simulink model "Boomerang_Simulink_Nav"  (R2023a)
settings: Solver=ode4  StartTime=0.0  StopTime=t  FixedStep=dt  MaxStep=maxstep  MinStep=minstep
values from neighbouring files (symbols this model uses):
  c = 5e-2    (= 0.05)    [Boomerang_Sim.m]
  CDdata = [x_CD, y_CD]    [Boomerang_Sim.m]
  CLdata = [x_CL, y_CL]    [Boomerang_Sim.m]
  CMdata = [x_CM, y_CM]    [Boomerang_Sim.m]
  Eul0 = [0; 0; 0]    [Boomerang_Sim.m]
  f = 1000    [Boomerang_Sim.m]
  g = 8.87    [Boomerang_Sim.m]
  invJ = inv(J)    [Boomerang_Sim.m]
  invTI0 = transpose(TI0)    [Boomerang_Sim.m]
  invTj = zeros(3,3,nw)    [Boomerang_Sim.m]
  J = J + (Ji(:,:,i))    [Boomerang_Sim.m]
  l_integrate = linspace(0,l_blade,n)    [Boomerang_Sim.m]
  m = m_b    (= 0.2)    [Boomerang_Sim.m]
  nw = 4    [Boomerang_Sim.m]
  omega0 = [0; 0; 10*pi*2]    [Boomerang_Sim.m]
  PHI0 = deg2rad(PHI0)    [Boomerang_Sim.m]
  PSI0 = deg2rad(PSI0)    [Boomerang_Sim.m]
  R_pos0 = [0; 0; 1.5]    [Boomerang_Sim.m]
  rho = 1.3288    [Boomerang_Sim.m]
  S = pi*R^2    (= 0.196349540849)    [Boomerang_Sim.m]
  THETA0 = deg2rad(THETA0)    [Boomerang_Sim.m]
  thetaj = 0    [Boomerang_Sim.m]
  TI0 = RI01*RI02*RI03    [Boomerang_Sim.m]
  Tj = zeros(3,3, nw)    [Boomerang_Sim.m]
  u0 = TI0*U0    [Boomerang_Sim.m]
  v_wind = [0; 0; 0]    [Boomerang_Sim.m]
  x_ac = zeros(3,nw)    [Boomerang_Sim.m]
undefined symbols (not defined in the file or in its folder): delta_theta, t_action
libraries: aerolibnav x2, simulink_extras x2
settings Model: Creator=dsantis  LastModifiedBy=dsantis

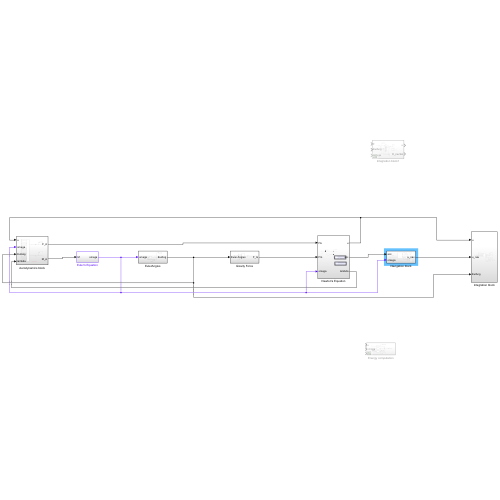
[thumbnail: Simulink's stored preview of the top-level diagram]
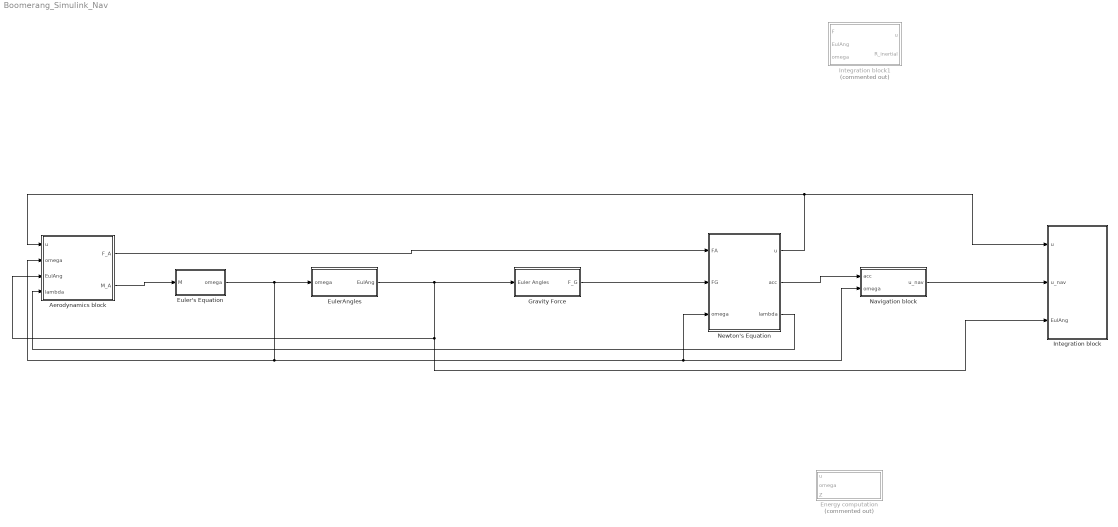
== system Boomerang_Simulink_Nav ==
  Aerodynamics block : Subsystem
  Energy computation : Subsystem  Commented=on
  Euler's Equation : Subsystem
  EulerAngles : Subsystem
  Gravity Force : Subsystem
  Integration block : Subsystem
  Integration block1 : Subsystem  Commented=on
  Navigation block : Subsystem
  Newton's Equation : Subsystem
  wires:
  Euler's Equation/1(omega) -> EulerAngles/1(omega), Aerodynamics block/2(omega), Newton's Equation/3(omega), Navigation block/2(omega)
  Newton's Equation/1(u) -> Aerodynamics block/1(u), Integration block/1(u)
  Gravity Force/1(F_G) -> Newton's Equation/2(FG)
  Aerodynamics block/2(M_A) -> Euler's Equation/1(M)
  EulerAngles/1(EulAng) -> Aerodynamics block/3(EulAng), Integration block/3(EulAng), Gravity Force/1(Euler Angles)
  Aerodynamics block/1(F_A) -> Newton's Equation/1(FA)
  Navigation block/1(u_nav) -> Integration block/2(u_nav)
  Newton's Equation/2(acc) -> Navigation block/1(acc)
  Newton's Equation/3(lambda) -> Aerodynamics block/4(lambda)

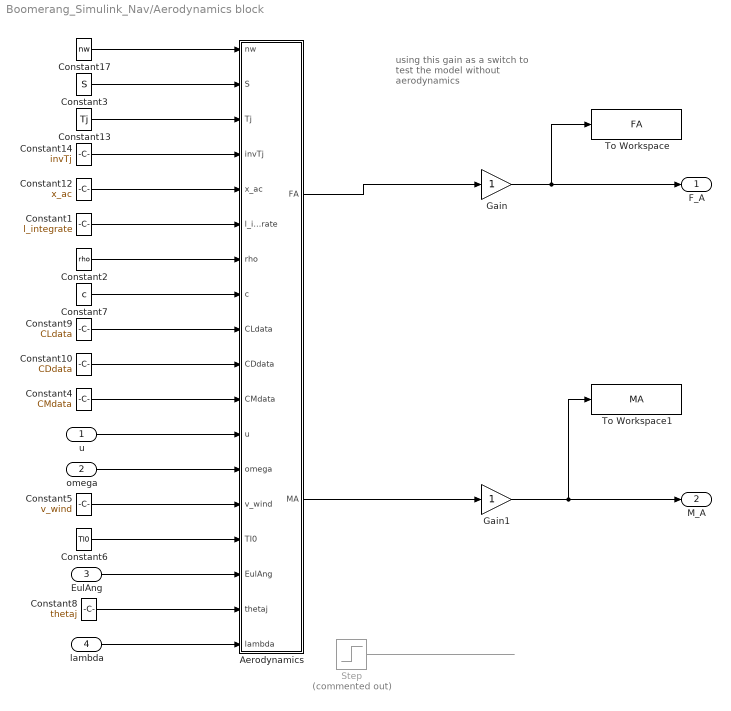
== system Boomerang_Simulink_Nav/Aerodynamics block ==
  note: using this gain as a switch
      | to test the model without aerodynamics
  u : Inport
  omega : Inport  Port=2
  EulAng : Inport  Port=3
  lambda : Inport  Port=4
  Aerodynamics : MATLAB Function  TreatAsAtomicUnit=on
  Constant1 : Constant  Value=l_integrate
  Constant10 : Constant  Value=CDdata
  Constant12 : Constant  Value=x_ac
  Constant13 : Constant  Value=Tj
  Constant14 : Constant  Value=invTj
  Constant17 : Constant  Value=nw
  Constant2 : Constant  Value=rho
  Constant3 : Constant  Value=S
  Constant4 : Constant  Value=CMdata
  Constant5 : Constant  Value=v_wind
  Constant6 : Constant  Value=TI0
  Constant7 : Constant  Value=c
  Constant8 : Constant  Value=thetaj
  Constant9 : Constant  Value=CLdata
  Gain : Gain
  Gain1 : Gain
  Step : Step  Commented=on  Time=t_action  After=delta_theta  SampleTime=0  VectorParams1D=off
  To Workspace : ToWorkspace  VariableName=FA  SampleTime=-1
  To Workspace1 : ToWorkspace  VariableName=MA  SampleTime=-1
  F_A : Outport
  M_A : Outport  Port=2
  wires:
  u/1 -> Aerodynamics/12(u)
  Constant2/1 -> Aerodynamics/7(rho)
  Constant9/1 -> Aerodynamics/9(CLdata)
  Constant10/1 -> Aerodynamics/10(CDdata)
  Constant1/1 -> Aerodynamics/6(l_integrate)
  Constant7/1 -> Aerodynamics/8(c)
  omega/1 -> Aerodynamics/13(omega)
  Constant12/1 -> Aerodynamics/5(x_ac)
  Constant14/1 -> Aerodynamics/4(invTj)
  Constant13/1 -> Aerodynamics/3(Tj)
  Aerodynamics/1(FA) -> Gain/1
  Constant17/1 -> Aerodynamics/1(nw)
  Constant3/1 -> Aerodynamics/2(S)
  Gain/1 -> To Workspace/1, F_A/1
  Constant4/1 -> Aerodynamics/11(CMdata)
  Step/1 -> ?
  Aerodynamics/2(MA) -> Gain1/1
  Constant5/1 -> Aerodynamics/14(v_wind)
  Constant6/1 -> Aerodynamics/15(TI0)
  EulAng/1 -> Aerodynamics/16(EulAng)
  Constant8/1 -> Aerodynamics/17(thetaj)
  lambda/1 -> Aerodynamics/18(lambda)
  Gain1/1 -> To Workspace1/1, M_A/1

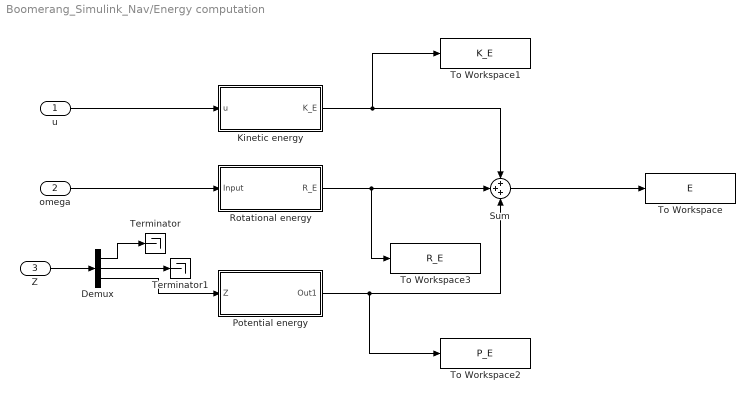
== system Boomerang_Simulink_Nav/Energy computation ==
  u : Inport
  omega : Inport  Port=2
  Z : Inport  Port=3
  Demux : Demux  Outputs=3
  Kinetic energy : Subsystem
  Potential energy : Subsystem
  Rotational energy : Subsystem
  Sum : Sum  Inputs=+++
  Terminator : Terminator
  Terminator1 : Terminator
  To Workspace : ToWorkspace  VariableName=E  SaveFormat=Timeseries  SampleTime=-1
  To Workspace1 : ToWorkspace  VariableName=K_E  SaveFormat=Timeseries  SampleTime=-1
  To Workspace2 : ToWorkspace  VariableName=P_E  SaveFormat=Timeseries  SampleTime=-1
  To Workspace3 : ToWorkspace  VariableName=R_E  SaveFormat=Timeseries  SampleTime=-1
  wires:
  u/1 -> Kinetic energy/1(u)
  omega/1 -> Rotational energy/1(Input)
  Z/1 -> Demux/1
  Demux/3 -> Potential energy/1(Z)
  Demux/1 -> Terminator/1
  Demux/2 -> Terminator1/1
  Kinetic energy/1(K_E) -> To Workspace1/1, Sum/1
  Rotational energy/1(R_E) -> To Workspace3/1, Sum/2
  Potential energy/1(Out1) -> To Workspace2/1, Sum/3
  Sum/1 -> To Workspace/1

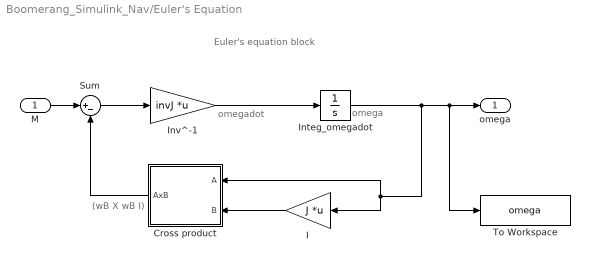
== system Boomerang_Simulink_Nav/Euler's Equation ==
  note: Euler's equation block
  note: (wB X wB I)
  note: omega
  note: omegadot
  M : Inport
  Cross product : Subsystem
  I : Gain  Gain=J  Multiplication=Matrix(K*u)
  Integ_omegadot : Integrator  InitialCondition=omega0
  Inv^-1 : Gain  Gain=invJ  Multiplication=Matrix(K*u) (u vector)
  Sum : Sum  Inputs=|+-
  To Workspace : ToWorkspace  VariableName=omega  SampleTime=-1
  omega : Outport  VectorParamsAs1DForOutWhenUnconnected=off
  wires:
  Integ_omegadot/1 -> To Workspace/1, omega/1, I/1, Cross product/1(A)
  I/1 -> Cross product/2(B)
  M/1 -> Sum/1
  Sum/1 -> Inv^-1/1
  Inv^-1/1 -> Integ_omegadot/1
  Cross product/1(AxB) -> Sum/2

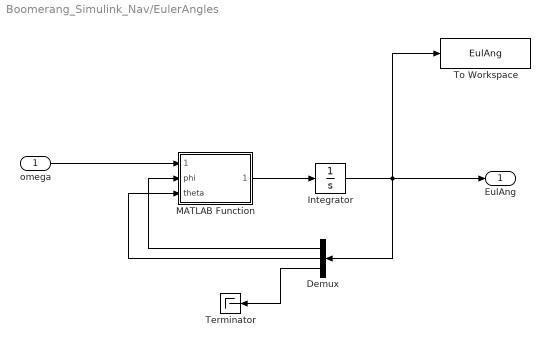
== system Boomerang_Simulink_Nav/EulerAngles ==
  omega : Inport
  Demux : Demux  Outputs=3
  Integrator : Integrator  InitialCondition=Eul0
  MATLAB Function : MATLAB Function  TreatAsAtomicUnit=on
  Terminator : Terminator
  To Workspace : ToWorkspace  VariableName=EulAng  SampleTime=-1
  EulAng : Outport
  wires:
  omega/1 -> MATLAB Function/1(omega)
  MATLAB Function/1(EulRate) -> Integrator/1
  Integrator/1 -> To Workspace/1, Demux/1, EulAng/1
  Demux/1 -> MATLAB Function/2(phi)
  Demux/2 -> MATLAB Function/3(theta)
  Demux/3 -> Terminator/1

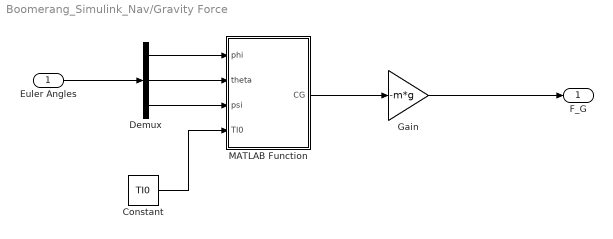
== system Boomerang_Simulink_Nav/Gravity Force ==
  Euler Angles : Inport
  Constant : Constant  Value=TI0
  Demux : Demux  Outputs=3
  Gain : Gain  Gain=-m*g
  MATLAB Function : MATLAB Function  TreatAsAtomicUnit=on
  F_G : Outport
  wires:
  Gain/1 -> F_G/1
  Demux/3 -> MATLAB Function/3(psi)
  Demux/2 -> MATLAB Function/2(theta)
  Demux/1 -> MATLAB Function/1(phi)
  MATLAB Function/1(CG) -> Gain/1
  Euler Angles/1 -> Demux/1
  Constant/1 -> MATLAB Function/4(TI0)

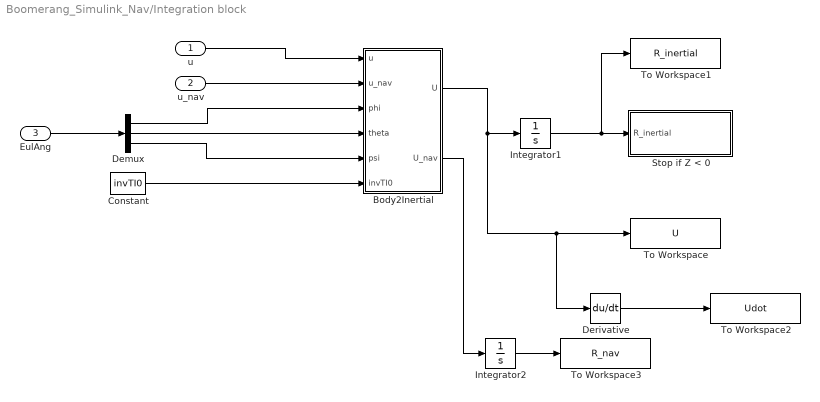
== system Boomerang_Simulink_Nav/Integration block ==
  u : Inport
  u_nav : Inport  Port=2
  EulAng : Inport  Port=3
  Body2Inertial : MATLAB Function  TreatAsAtomicUnit=on
  Constant : Constant  Value=invTI0
  Demux : Demux  Outputs=3
  Derivative : Derivative
  Integrator1 : Integrator  InitialCondition=R_pos0
  Integrator2 : Integrator  InitialCondition=R_pos0
  Stop if Z < 0 : Subsystem
  To Workspace : ToWorkspace  VariableName=U  SampleTime=-1
  To Workspace1 : ToWorkspace  VariableName=R_inertial  SampleTime=-1
  To Workspace2 : ToWorkspace  VariableName=Udot  SaveFormat=Timeseries  SampleTime=-1
  To Workspace3 : ToWorkspace  VariableName=R_nav  SampleTime=-1
  wires:
  Derivative/1 -> To Workspace2/1
  Integrator1/1 -> Stop if Z < 0/1(R_inertial), To Workspace1/1
  Body2Inertial/1(U) -> Derivative/1, To Workspace/1, Integrator1/1
  Demux/3 -> Body2Inertial/5(psi)
  Demux/2 -> Body2Inertial/4(theta)
  u/1 -> Body2Inertial/1(u)
  Demux/1 -> Body2Inertial/3(phi)
  Constant/1 -> Body2Inertial/6(invTI0)
  EulAng/1 -> Demux/1
  u_nav/1 -> Body2Inertial/2(u_nav)
  Body2Inertial/2(U_nav) -> Integrator2/1
  Integrator2/1 -> To Workspace3/1

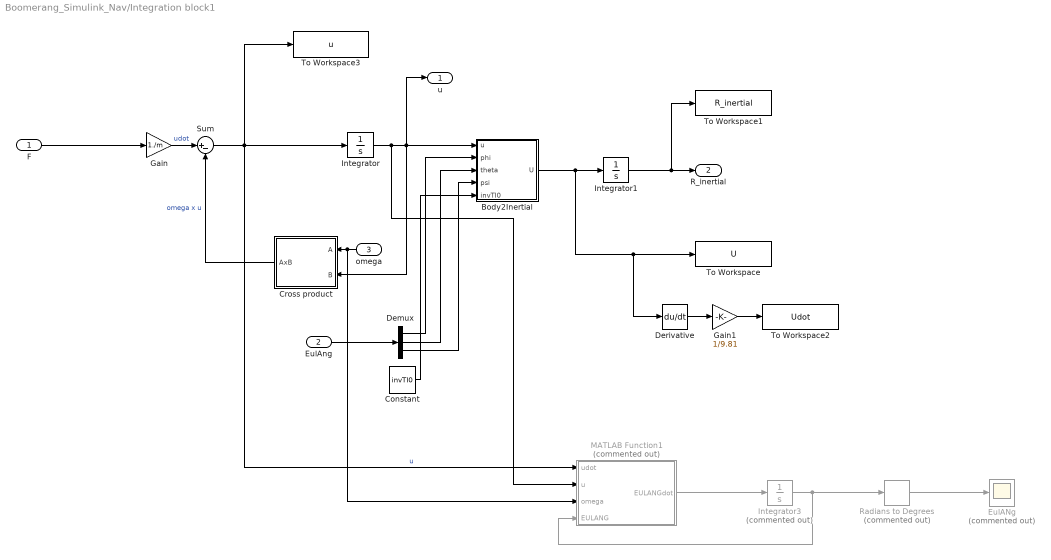
== system Boomerang_Simulink_Nav/Integration block1 ==
  F : Inport
  EulAng : Inport  Port=2
  omega : Inport  Port=3
  Body2Inertial : MATLAB Function  TreatAsAtomicUnit=on
  Constant : Constant  Value=invTI0
  Cross product : Subsystem
  Demux : Demux  Outputs=3
  Derivative : Derivative
  EulANg : Scope  Commented=on
  Gain : Gain  Gain=1./m
  Gain1 : Gain  Gain=1/9.81
  Integrator : Integrator  InitialCondition=u0
  Integrator1 : Integrator  InitialCondition=R_pos0
  Integrator3 : Integrator  Commented=on  InitialCondition=[PHI0; THETA0; PSI0]
  MATLAB Function1 : MATLAB Function  Commented=on  TreatAsAtomicUnit=on
  Radians to Degrees : simulink_extras/Transformations/Radians to Degrees  Commented=on
  Sum : Sum  Inputs=|+-
  To Workspace : ToWorkspace  VariableName=U  SampleTime=-1
  To Workspace1 : ToWorkspace  VariableName=R_inertial  SampleTime=-1
  To Workspace2 : ToWorkspace  VariableName=Udot  SaveFormat=Timeseries  SampleTime=-1
  To Workspace3 : ToWorkspace  VariableName=u  SampleTime=-1
  u : Outport
  R_inertial : Outport  Port=2
  wires:
  Cross product/1(AxB) -> Sum/2  "omega x u"
  Integrator/1 -> Cross product/2(B), Body2Inertial/1(u), u/1, MATLAB Function1/2(u)
  Integrator1/1 -> To Workspace1/1, R_inertial/1
  Gain/1 -> Sum/1  "udot"
  EulAng/1 -> Demux/1
  Demux/1 -> Body2Inertial/2(phi)
  Demux/2 -> Body2Inertial/3(theta)
  Demux/3 -> Body2Inertial/4(psi)
  Constant/1 -> Body2Inertial/5(invTI0)
  F/1 -> Gain/1
  Body2Inertial/1(U) -> Derivative/1, To Workspace/1, Integrator1/1
  Sum/1 -> To Workspace3/1, MATLAB Function1/1(udot), Integrator/1  "u"
  MATLAB Function1/1(EULANGdot) -> Integrator3/1
  Integrator3/1 -> Radians to Degrees/1, MATLAB Function1/4(EULANG)
  Radians to Degrees/1 -> EulANg/1
  Derivative/1 -> Gain1/1
  Gain1/1 -> To Workspace2/1
  omega/1 -> MATLAB Function1/3(omega), Cross product/1(A)

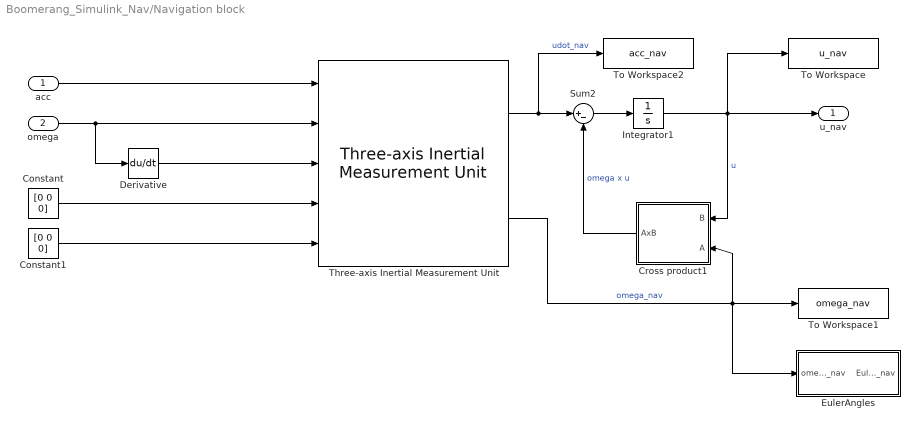
== system Boomerang_Simulink_Nav/Navigation block ==
  acc : Inport
  omega : Inport  Port=2
  Constant : Constant  Value=[0 0 0]
  Constant1 : Constant  Value=[0 0 0]
  Cross product1 : Subsystem
  Derivative : Derivative
  EulerAngles : Subsystem
  Integrator1 : Integrator  InitialCondition=u0
  Sum2 : Sum  Inputs=|+-
  Three-axis Inertial Measurement Unit : aerolibnav/Three-axis Inertial Measurement Unit  units=Metric (MKS)  imu=[0 0 0]  i_Ts=1/f  dtype_a=off  w_a=190  z_a=0.707  a_sf_cc=acc.sf  a_bias=acc.bias  a_sat=acc.lim  dtype_g=off  w_g=190  z_g=0.707  g_sf_cc=gyro.sf  g_bias=gyro.bias  g_sens=gyro.gbias  g_sat=gyro.lim  i_rand=on  i_seeds=[23093 23094 23095 23096 23097 23098]  i_pow=noise
  To Workspace : ToWorkspace  VariableName=u_nav  SampleTime=-1
  To Workspace1 : ToWorkspace  VariableName=omega_nav  SampleTime=-1
  To Workspace2 : ToWorkspace  VariableName=acc_nav  SampleTime=-1
  u_nav : Outport
  wires:
  Constant1/1 -> Three-axis Inertial Measurement Unit/5
  Derivative/1 -> Three-axis Inertial Measurement Unit/3
  Cross product1/1(AxB) -> Sum2/2  "omega x u"
  Sum2/1 -> Integrator1/1
  Constant/1 -> Three-axis Inertial Measurement Unit/4
  Three-axis Inertial Measurement Unit/2 -> EulerAngles/1(omega_nav), To Workspace1/1, Cross product1/2(A)  "omega_nav"
  acc/1 -> Three-axis Inertial Measurement Unit/1
  Integrator1/1 -> Cross product1/1(B), u_nav/1, To Workspace/1  "u"
  Three-axis Inertial Measurement Unit/1 -> To Workspace2/1, Sum2/1  "udot_nav"
  omega/1 -> Derivative/1, Three-axis Inertial Measurement Unit/2

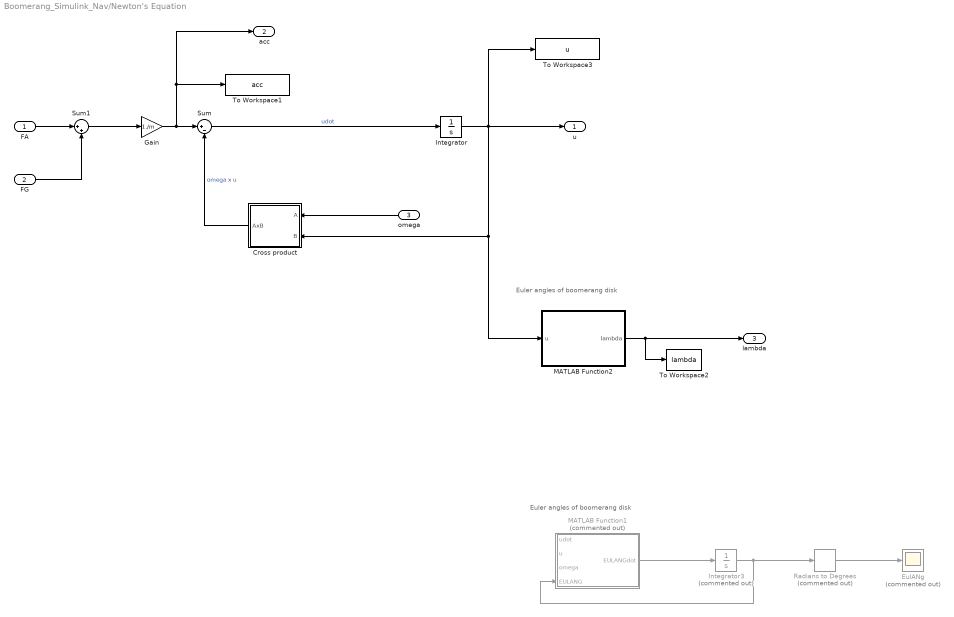
== system Boomerang_Simulink_Nav/Newton's Equation ==
  note: Euler angles of boomerang disk
  note: Euler angles of boomerang disk
  FA : Inport
  FG : Inport  Port=2
  omega : Inport  Port=3
  Cross product : Subsystem
  EulANg : Scope  Commented=on
  Gain : Gain  Gain=1./m
  Integrator : Integrator  InitialCondition=u0
  Integrator3 : Integrator  Commented=on  InitialCondition=[PHI0; THETA0; PSI0]
  MATLAB Function1 : MATLAB Function  Commented=on  TreatAsAtomicUnit=on
  MATLAB Function2 : MATLAB Function  TreatAsAtomicUnit=on
  Radians to Degrees : simulink_extras/Transformations/Radians to Degrees  Commented=on
  Sum : Sum  Inputs=|+-
  Sum1 : Sum  Inputs=|++
  To Workspace1 : ToWorkspace  VariableName=acc  SampleTime=-1
  To Workspace2 : ToWorkspace  VariableName=lambda  SampleTime=-1
  To Workspace3 : ToWorkspace  VariableName=u  SampleTime=-1
  u : Outport
  acc : Outport  Port=2
  lambda : Outport  Port=3
  wires:
  Cross product/1(AxB) -> Sum/2  "omega x u"
  Gain/1 -> acc/1, To Workspace1/1, Sum/1
  FA/1 -> Sum1/1
  Sum/1 -> Integrator/1  "udot"
  MATLAB Function1/1(EULANGdot) -> Integrator3/1
  Integrator3/1 -> Radians to Degrees/1, MATLAB Function1/4(EULANG)
  Radians to Degrees/1 -> EulANg/1
  omega/1 -> Cross product/1(A)
  FG/1 -> Sum1/2
  Sum1/1 -> Gain/1
  MATLAB Function2/1(lambda) -> lambda/1, To Workspace2/1
  Integrator/1 -> MATLAB Function2/1(u), Cross product/2(B), To Workspace3/1, u/1

== system Boomerang_Simulink_Nav/Energy computation/Kinetic energy ==
  u : Inport
  Gain : Gain  Gain=0.5*m
  Norm : MATLAB Function  TreatAsAtomicUnit=on
  K_E : Outport
  wires:
  u/1 -> Norm/1(u)
  Norm/1(y) -> Gain/1
  Gain/1 -> K_E/1

== system Boomerang_Simulink_Nav/Energy computation/Potential energy ==
  Z : Inport
  Gain : Gain  Gain=m*g
  Out1 : Outport
  wires:
  Z/1 -> Gain/1
  Gain/1 -> Out1/1

== system Boomerang_Simulink_Nav/Energy computation/Rotational energy ==
  Input : Inport
  Dot Product : DotProduct  OutDataTypeStr=Inherit: Inherit via internal rule
  Gain : Gain  Gain=0.5*J  Multiplication=Matrix(u*K)
  R_E : Outport
  wires:
  Input/1 -> Dot Product/2, Gain/1
  Gain/1 -> Dot Product/1
  Dot Product/1 -> R_E/1

== system Boomerang_Simulink_Nav/Euler's Equation/Cross product ==
  A : Inport
  B : Inport  Port=2
  MATLAB Fcn : MATLABFcn  MATLABFcn=cross(u(1:3),u(4:6))
  Mux : Mux  Inputs=2
  AxB : Outport  VectorParamsAs1DForOutWhenUnconnected=off
  wires:
  A/1 -> Mux/1
  B/1 -> Mux/2
  Mux/1 -> MATLAB Fcn/1
  MATLAB Fcn/1 -> AxB/1

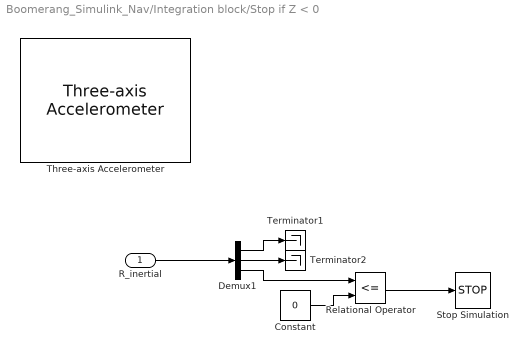
== system Boomerang_Simulink_Nav/Integration block/Stop if Z < 0 ==
  R_inertial : Inport
  Constant : Constant  Value=0
  Demux1 : Demux  Outputs=3
  Relational Operator : RelationalOperator  Operator=<=  OutDataTypeStr=boolean  RndMeth=Simplest  InputSameDT=off
  Stop Simulation : Stop
  Terminator1 : Terminator
  Terminator2 : Terminator
  Three-axis Accelerometer : aerolibnav/Three-axis Accelerometer  units=Metric (MKS)  acc=[0 0 0]  gtype=on  dtype_a=on  w_a=190  z_a=0.707  a_sf_cc=[1 0 0; 0 1 0; 0 0 1]  a_bias=[0 0 0]  a_Ts=0  a_rand=on  a_seeds=[23093 23094 23095]  a_pow=[0.001 0.001 0.001]  a_sat="[-inf  -inf  -inf  inf inf inf]"
  wires:
  R_inertial/1 -> Demux1/1
  Demux1/1 -> Terminator1/1
  Demux1/3 -> Relational Operator/1
  Demux1/2 -> Terminator2/1
  Constant/1 -> Relational Operator/2
  Relational Operator/1 -> Stop Simulation/1

== system Boomerang_Simulink_Nav/Integration block1/Cross product ==
  A : Inport
  B : Inport  Port=2
  MATLAB Fcn : MATLABFcn  MATLABFcn=cross(u(1:3),u(4:6))
  Mux : Mux  Inputs=2
  AxB : Outport  VectorParamsAs1DForOutWhenUnconnected=off
  wires:
  A/1 -> Mux/1
  B/1 -> Mux/2
  Mux/1 -> MATLAB Fcn/1
  MATLAB Fcn/1 -> AxB/1

== system Boomerang_Simulink_Nav/Navigation block/Cross product1 ==
  B : Inport
  A : Inport  Port=2
  MATLAB Fcn : MATLABFcn  MATLABFcn=cross(u(1:3),u(4:6))
  Mux : Mux  Inputs=2
  AxB : Outport  VectorParamsAs1DForOutWhenUnconnected=off
  wires:
  A/1 -> Mux/1
  B/1 -> Mux/2
  Mux/1 -> MATLAB Fcn/1
  MATLAB Fcn/1 -> AxB/1

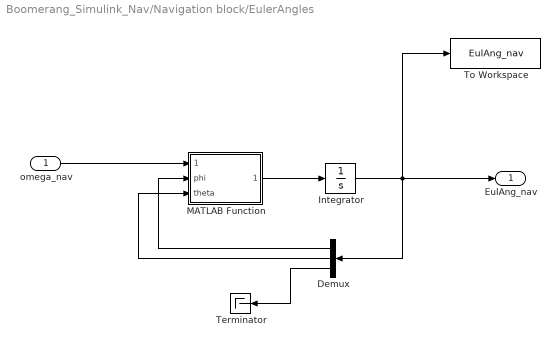
== system Boomerang_Simulink_Nav/Navigation block/EulerAngles ==
  omega_nav : Inport
  Demux : Demux  Outputs=3
  Integrator : Integrator  InitialCondition=Eul0
  MATLAB Function : MATLAB Function  TreatAsAtomicUnit=on
  Terminator : Terminator
  To Workspace : ToWorkspace  VariableName=EulAng_nav  SampleTime=-1
  EulAng_nav : Outport
  wires:
  omega_nav/1 -> MATLAB Function/1(omega)
  MATLAB Function/1(EulRate) -> Integrator/1
  Integrator/1 -> To Workspace/1, Demux/1, EulAng_nav/1
  Demux/1 -> MATLAB Function/2(phi)
  Demux/2 -> MATLAB Function/3(theta)
  Demux/3 -> Terminator/1

== system Boomerang_Simulink_Nav/Newton's Equation/Cross product ==
  A : Inport
  B : Inport  Port=2
  MATLAB Fcn : MATLABFcn  MATLABFcn=cross(u(1:3),u(4:6))
  Mux : Mux  Inputs=2
  AxB : Outport  VectorParamsAs1DForOutWhenUnconnected=off
  wires:
  A/1 -> Mux/1
  B/1 -> Mux/2
  Mux/1 -> MATLAB Fcn/1
  MATLAB Fcn/1 -> AxB/1

== matlab function Boomerang_Simulink_Nav/Integration block1/Body2Inertial ==
  data: u input; U output; phi input; theta input; psi input; invTI0 input
function U = fcn(u, phi, theta, psi, invTI0)
R01 = [
    1, 0, 0;
    0, cos(phi), sin(phi);
    0, -sin(phi), cos(phi)
    ];
R02 = [
    cos(theta), 0, -sin(theta);
    0, 1, 0;
    sin(theta), 0, cos(theta)
];
R03 = [
    cos(psi), sin(psi), 0;
    -sin(psi), cos(psi), 0;
    0, 0, 1
];
T0 = R01*R02*R03;
invT0 = transpose(T0);
U = invTI0*invT0*u;

== matlab function Boomerang_Simulink_Nav/Newton's Equation/MATLAB Function1 ==
  data: udot input; u input; EULANGdot output; omega input; EULANG input
function EULANGdot = fcn(udot, u, omega, EULANG)
udotx = udot(1);
udoty = udot(2);

ux = u(1);
uy = u(2);

p = omega(1);
q = omega(2);
r = omega(3);

PHI = EULANG(1);
THETA = EULANG(2);

rn = r + (udoty*ux - udotx*uy)/(ux^2 + uy^2);
lambda = -tan(uy/ux);

PHIdot = (p*cos(lambda) - q*sin(lambda)) + (p*sin(lambda) + q*cos(lambda))*sin(PHI)*tan(THETA) + ...
    rn*cos(PHI)*tan(THETA);
THETAdot = (p*sin(lambda) + q*cos(lambda))*cos(PHI) - rn*sin(PHI);
PSIdot = (p*sin(lambda) + q*cos(lambda))*sin(PHI)/cos(THETA) + rn*cos(PHI)/cos(THETA);

EULANGdot = [PHIdot; THETAdot; PSIdot];

== matlab function Boomerang_Simulink_Nav/Integration block1/MATLAB Function1 ==
  data: udot input; u input; EULANGdot output; omega input; EULANG input
function EULANGdot = fcn(udot, u, omega, EULANG)
udotx = udot(1);
udoty = udot(2);

ux = u(1);
uy = u(2);

p = omega(1);
q = omega(2);
r = omega(3);

PHI = EULANG(1);
THETA = EULANG(2);

rn = r + (udoty*ux - udotx*uy)/(ux^2 + uy^2);
lambda = -tan(uy/ux);

PHIdot = (p*cos(lambda) - q*sin(lambda)) + (p*sin(lambda) + q*cos(lambda))*sin(PHI)*tan(THETA) + ...
    rn*cos(PHI)*tan(THETA);
THETAdot = (p*sin(lambda) + q*cos(lambda))*cos(PHI) - rn*sin(PHI);
PSIdot = (p*sin(lambda) + q*cos(lambda))*sin(PHI)/cos(THETA) + rn*cos(PHI)/cos(THETA);

EULANGdot = [PHIdot; THETAdot; PSIdot];

== matlab function Boomerang_Simulink_Nav/Newton's Equation/MATLAB Function2 ==
  data: u input; lambda output
function lambda  = fcn(u)
% udotx = udot(1);
% udoty = udot(2);

ux = u(1);
uy = u(2);

% p = omega(1);
% q = omega(2);
% r = omega(3);
% 
% PHI = EULANG(1);
% THETA = EULANG(2);
% 
% rn = r + (udoty*ux - udotx*uy)/(ux^2 + uy^2);

lambda = -atan2(uy,ux);

% PHIdot = (p*cos(lambda) - q*sin(lambda)) + (p*sin(lambda) + q*cos(lambda))*sin(PHI)*tan(THETA) + ...
%     rn*cos(PHI)*tan(THETA);
% THETAdot = (p*sin(lambda) + q*cos(lambda))*cos(PHI) - rn*sin(PHI);
% PSIdot = (p*sin(lambda) + q*cos(lambda))*sin(PHI)/cos(THETA) + rn*cos(PHI)/cos(THETA);

% EULANGdot = [PHIdot; THETAdot; PSIdot];

== matlab function Boomerang_Simulink_Nav/Navigation block/EulerAngles/MATLAB Function ==
  data: omega input; EulRate output; phi input; theta input
function EulRate = fcn(omega, phi, theta)

phidot = omega(1) + omega(2)*sin(phi)*tan(theta) + omega(3)*cos(phi)*tan(theta);
thetadot = omega(2)*cos(phi) - omega(3)*sin(phi);
psidot = omega(2)*sin(phi)/cos(theta) + omega(3)*cos(phi)/cos(theta);

EulRate = [phidot; thetadot; psidot];

== matlab function Boomerang_Simulink_Nav/Aerodynamics block/Aerodynamics ==
  settings: updateMethod=DISCRETE
  data: nw input; S input; Tj input; invTj input; x_ac input; l_integrate input; rho input; c input; CLdata input; CDdata input; CMdata input; u input; omega input; v_wind input; TI0 input; EulAng input; FA output; thetaj input; MA output; lambda input
function [FA, MA] = fcn(nw, S, Tj, invTj, x_ac, l_integrate, rho, c, CLdata, CDdata, CMdata,u, omega, v_wind, TI0, EulAng, thetaj, lambda)

phi = EulAng(1);
theta = EulAng(2);
psi = EulAng(3);
gamma = deg2rad(90);

R01 = [1, 0, 0; 0, cos(phi), sin(phi); 0, -sin(phi), cos(phi)];
R02 = [cos(theta), 0, -sin(theta); 0, 1, 0; sin(theta), 0, cos(theta)];
R03 = [cos(psi), sin(psi), 0; -sin(psi), cos(psi), 0; 0, 0, 1];
T0 = R01*R02*R03;

persistent flag v_bar
if isempty(flag)
    flag = false;
    v_bar = 0;
end
r = l_integrate./l_integrate(end);

% Piecewise linear fit for CL
C_L = @(alpha) interp1(CLdata(:,1), CLdata(:,2), alpha, 'linear', 'extrap');

% Piecewise linear fit for CD
C_D = @(alpha) interp1(CDdata(:,1), CDdata(:,2), alpha, 'linear', 'extrap');

 % Piecewise linear fit for CM
C_M = @(alpha) interp1(CMdata(:,1), CMdata(:,2), alpha, 'linear', 'extrap');

FA = [0; 0; 0];
MA = [0;0;0];

n = length(l_integrate);

for i = 1:nw
    % Computing induced velocity considering linear variation along the
    % longitudinal direction
    kx = 1.5;
    v_ind = [zeros(size(l_integrate)), zeros(size(l_integrate)), v_bar*(1+kx*cos(lambda + gamma*(i-1))*r)]';

    rA = x_ac(:,i).*ones(3,n) + invTj(:,:,i)*[zeros(1,n); l_integrate'; zeros(1,n)];
    
    w = Tj(:,:,i)*( (-u -cross(omega.*ones(3,n), rA)) + v_ind + T0*TI0*v_wind);
    alpha = (atan2(w(3,:),w(1,:))) + thetaj;
    
    % Computing the tip-loss factor F
    f = abs(nw/2.*(1-r')./(r'.*alpha));
    F =2/pi*acos(exp(-f));
    w2 = w(1,:).^2 + w(3,:).^2;
    
    l = (0.5*rho*c).*w2.*C_L(alpha);
    d = (0.5*rho*c).*w2.*C_D(alpha);
    m_eta = (0.5*rho*c^2).*w2.*C_M(alpha);

    int_funx = F.*(-l.*sin(alpha) + d.*cos(alpha));
    int_funz = (l.*cos(alpha) + d.*sin(alpha));
    
    % int_funMx = (l.*cos(alpha) + d.*sin(alpha)).*l_integrate';
    funM = cross([zeros(1,n); l_integrate'; zeros(1,n)], [int_funx; zeros(1,n); int_funz]);
    int_funMx = funM(1,:);
    int_funMy = m_eta; 
    int_funMz = funM(3,:);
 
    FxjA = trapz(l_integrate,int_funx);
    FzjA = trapz(l_integrate,int_funz);

    MxjA = trapz(l_integrate,int_funMx);
    MyjA = trapz(l_integrate,int_funMy);
    MzjA = trapz(l_integrate,int_funMz);

    FjA = [FxjA; 0; FzjA];
    FA = FA + invTj(:,:,i)*FjA;

    MjA = [MxjA'; MyjA; MzjA];
    MA = MA + invTj(:,:,i)*MjA + cross(x_ac(:,i), invTj(:,:,i)*FjA);
end
f = @(v_ind) v_ind - FA(3)/(2*rho*S*sqrt(norm([u(1) u(2)])^2 + (u(3)-v_ind)^2));
v_bar = fzero(f,0);

== matlab function Boomerang_Simulink_Nav/Gravity Force/MATLAB Function ==
  data: phi input; theta input; psi input; CG output; TI0 input
function CG = fcn(phi, theta, psi, TI0)
R01 = [
    1, 0, 0;
    0, cos(phi), sin(phi);
    0, -sin(phi), cos(phi)
    ];
R02 = [
    cos(theta), 0, -sin(theta);
    0, 1, 0;
    sin(theta), 0, cos(theta)
];
R03 = [
    cos(psi), sin(psi), 0;
    -sin(psi), cos(psi), 0;
    0, 0, 1
];
T0 = R01*R02*R03;

CG = T0*TI0*[0; 0; 1];

== matlab function Boomerang_Simulink_Nav/Integration block/Body2Inertial ==
  data: u input; u_nav input; U output; phi input; theta input; psi input; invTI0 input; U_nav output
function [U, U_nav] = fcn(u, u_nav, phi, theta, psi, invTI0)
R01 = [
    1, 0, 0;
    0, cos(phi), sin(phi);
    0, -sin(phi), cos(phi)
    ];
R02 = [
    cos(theta), 0, -sin(theta);
    0, 1, 0;
    sin(theta), 0, cos(theta)
];
R03 = [
    cos(psi), sin(psi), 0;
    -sin(psi), cos(psi), 0;
    0, 0, 1
];
T0 = R01*R02*R03;
invT0 = transpose(T0);

U = invTI0*invT0*u;
U_nav = invTI0*invT0*u_nav;

== matlab function Boomerang_Simulink_Nav/EulerAngles/MATLAB Function ==
  data: omega input; EulRate output; phi input; theta input
function EulRate = fcn(omega, phi, theta)

phidot = omega(1) + omega(2)*sin(phi)*tan(theta) + omega(3)*cos(phi)*tan(theta);
thetadot = omega(2)*cos(phi) - omega(3)*sin(phi);
psidot = omega(2)*sin(phi)/cos(theta) + omega(3)*cos(phi)/cos(theta);

EulRate = [phidot; thetadot; psidot];

== matlab function Boomerang_Simulink_Nav/Energy computation/Kinetic energy/Norm ==
  data: u input; y output
function y = fcn(u)

y = norm(u)^2;
